simulink model "ac3_example_MMCT"  (R2023a)
settings: Solver=FixedStepDiscrete  StartTime=0.0  StopTime=3  FixedStep=Ts  RelTol=1e-3  EnableMultiTasking=on
PreLoadFcn:
  | Ts = 2e-6;
undefined symbols (not defined in the file): DiscIntNeverNeededParam
libraries: simulink_extras x7, spsCurrentMeasurementLib x3, spsVoltageMeasurementLib x3, spsDrivesPrivateModels x2, spsStairGeneratorLib x2, spsThreePhaseSourceLib x1, spsDrivesDcBusModel x1, spsSpaceVectorModulatorLib x1, eeAdaptiveController x1, slctrlblks x1, simulink x1, slpidlib x1
(part 3 of 3)

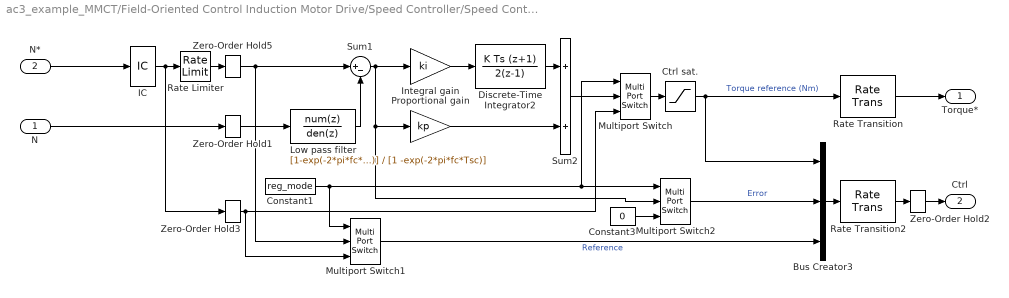
== system ac3_example_MMCT/Field-Oriented Control Induction Motor Drive/Speed Controller/Speed Controller (AC)/AC678/AC678 ==
  N : Inport
  N* : Inport  Port=2
  Bus Creator3 : BusCreator  Inputs=3
  Constant1 : Constant  Value=reg_mode
  Constant3 : Constant  Value=0
  Ctrl sat. : Saturate  UpperLimit=ctrl_sat(2)  LowerLimit=ctrl_sat(1)
  Discrete-Time Integrator2 : DiscreteIntegrator  IntegratorMethod=Integration: Trapezoidal  SampleTime=Tsc  LimitOutput=on  UpperSaturationLimit=ctrl_sat(2)  LowerSaturationLimit=ctrl_sat(1)  ICPrevOutput=DiscIntNeverNeededParam  ICPrevScaledInput=DiscIntNeverNeededParam
  IC : InitialCondition  Value=0
  Integral gain : Gain  Gain=ki  SaturateOnIntegerOverflow=on  OutDataTypeStr=Inherit: Same as input  ParamDataTypeStr=Inherit: Same as input
  Low pass filter : DiscreteTransferFcn  Numerator=[1-exp(-2*pi*fc*Tsc)]  Denominator=[1 -exp(-2*pi*fc*Tsc)]  SampleTime=Tsc
  Multiport Switch : MultiPortSwitch  Inputs=2  InputSameDT=off
  Multiport Switch1 : MultiPortSwitch  Inputs=2  InputSameDT=off
  Multiport Switch2 : MultiPortSwitch  Inputs=2  InputSameDT=off
  Proportional gain : Gain  Gain=kp  SaturateOnIntegerOverflow=on  OutDataTypeStr=Inherit: Same as input  ParamDataTypeStr=Inherit: Same as input
  Rate Limiter : RateLimiter  RisingSlewLimit=ramp(2)  FallingSlewLimit=ramp(1)  SampleTimeMode=inherited  LinearizeAsGain=off
  Rate Transition : RateTransition
  Rate Transition2 : RateTransition
  Sum1 : Sum  Inputs=|+-  InputSameDT=on  SaturateOnIntegerOverflow=on  OutDataTypeStr=Inherit: Same as first input
  Sum2 : Sum  InputSameDT=on  SaturateOnIntegerOverflow=on  OutDataTypeStr=Inherit: Same as first input
  Zero-Order Hold1 : ZeroOrderHold  SampleTime=Tsc
  Zero-Order Hold2 : ZeroOrderHold  SampleTime=Ts
  Zero-Order Hold3 : ZeroOrderHold  SampleTime=Tsc
  Zero-Order Hold5 : ZeroOrderHold  SampleTime=Tsc
  Torque* : Outport  VectorParamsAs1DForOutWhenUnconnected=off
  Ctrl : Outport  Port=2  VectorParamsAs1DForOutWhenUnconnected=off
  wires:
  N/1 -> Zero-Order Hold1/1
  N*/1 -> IC/1
  Ctrl sat./1 -> Rate Transition/1, Bus Creator3/1  "Torque reference (Nm)"
  Integral gain/1 -> Discrete-Time Integrator2/1
  Sum1/1 -> Integral gain/1, Proportional gain/1, Multiport Switch2/2
  Discrete-Time Integrator2/1 -> Sum2/1
  Proportional gain/1 -> Sum2/2
  Rate Transition/1 -> Torque*/1
  IC/1 -> Rate Limiter/1, Zero-Order Hold3/1
  Zero-Order Hold1/1 -> Low pass filter/1
  Rate Transition2/1 -> Zero-Order Hold2/1
  Bus Creator3/1 -> Rate Transition2/1
  Zero-Order Hold2/1 -> Ctrl/1
  Low pass filter/1 -> Sum1/2
  Rate Limiter/1 -> Zero-Order Hold5/1
  Zero-Order Hold5/1 -> Sum1/1, Multiport Switch1/2
  Multiport Switch/1 -> Ctrl sat./1
  Constant1/1 -> Multiport Switch2/1, Multiport Switch/1, Multiport Switch1/1
  Sum2/1 -> Multiport Switch/2
  Zero-Order Hold3/1 -> Multiport Switch/3, Multiport Switch1/3
  Multiport Switch1/1 -> Bus Creator3/3  "Reference"
  Multiport Switch2/1 -> Bus Creator3/2  "Error"
  Constant3/1 -> Multiport Switch2/3

== system ac3_example_MMCT/Field-Oriented Control Induction Motor Drive/F.O.C./Detailed/Switching control/Control 1-2/Subsystem1 ==
  Sig : Inport
  Constant : Constant
  Constant1 : Constant  Value=freq_max
  Discrete-Time Integrator : DiscreteIntegrator  IntegratorMethod=Integration: Trapezoidal  ExternalReset=rising  SampleTime=Tvect  ICPrevOutput=DiscIntNeverNeededParam  ICPrevScaledInput=DiscIntNeverNeededParam
  Relational Operator : RelationalOperator  ZeroCross=off  InputSameDT=off
  Unit Delay : UnitDelay  SampleTime=Tvect  HasFrameUpgradeWarning=on
  Trig : Outport  VectorParamsAs1DForOutWhenUnconnected=off
  wires:
  Constant1/1 -> Discrete-Time Integrator/1
  Constant/1 -> Relational Operator/2
  Discrete-Time Integrator/1 -> Relational Operator/1
  Relational Operator/1 -> Unit Delay/1
  Sig/1 -> Discrete-Time Integrator/2
  Unit Delay/1 -> Trig/1

== system ac3_example_MMCT/Field-Oriented Control Induction Motor Drive/F.O.C./Detailed/Switching control/Control 1-2/Subsystem3 ==
  Sig : Inport
  Constant : Constant
  Constant1 : Constant  Value=freq_max
  Discrete-Time Integrator : DiscreteIntegrator  IntegratorMethod=Integration: Trapezoidal  ExternalReset=rising  SampleTime=Tvect  ICPrevOutput=DiscIntNeverNeededParam  ICPrevScaledInput=DiscIntNeverNeededParam
  Relational Operator : RelationalOperator  ZeroCross=off  InputSameDT=off
  Unit Delay : UnitDelay  SampleTime=Tvect  HasFrameUpgradeWarning=on
  Trig : Outport  VectorParamsAs1DForOutWhenUnconnected=off
  wires:
  Unit Delay/1 -> Trig/1
  Sig/1 -> Discrete-Time Integrator/2
  Relational Operator/1 -> Unit Delay/1
  Discrete-Time Integrator/1 -> Relational Operator/1
  Constant/1 -> Relational Operator/2
  Constant1/1 -> Discrete-Time Integrator/1

== system ac3_example_MMCT/Field-Oriented Control Induction Motor Drive/F.O.C./Detailed/Switching control/Control 3-4/Subsystem1 ==
  Sig : Inport
  Constant : Constant
  Constant1 : Constant  Value=freq_max
  Discrete-Time Integrator : DiscreteIntegrator  IntegratorMethod=Integration: Trapezoidal  ExternalReset=rising  SampleTime=Tvect  ICPrevOutput=DiscIntNeverNeededParam  ICPrevScaledInput=DiscIntNeverNeededParam
  Relational Operator : RelationalOperator  ZeroCross=off  InputSameDT=off
  Unit Delay : UnitDelay  SampleTime=Tvect  HasFrameUpgradeWarning=on
  Trig : Outport  VectorParamsAs1DForOutWhenUnconnected=off
  wires:
  Unit Delay/1 -> Trig/1
  Sig/1 -> Discrete-Time Integrator/2
  Relational Operator/1 -> Unit Delay/1
  Discrete-Time Integrator/1 -> Relational Operator/1
  Constant/1 -> Relational Operator/2
  Constant1/1 -> Discrete-Time Integrator/1

== system ac3_example_MMCT/Field-Oriented Control Induction Motor Drive/F.O.C./Detailed/Switching control/Control 3-4/Subsystem3 ==
  Sig : Inport
  Constant : Constant
  Constant1 : Constant  Value=freq_max
  Discrete-Time Integrator : DiscreteIntegrator  IntegratorMethod=Integration: Trapezoidal  ExternalReset=rising  SampleTime=Tvect  ICPrevOutput=DiscIntNeverNeededParam  ICPrevScaledInput=DiscIntNeverNeededParam
  Relational Operator : RelationalOperator  ZeroCross=off  InputSameDT=off
  Unit Delay : UnitDelay  SampleTime=Tvect  HasFrameUpgradeWarning=on
  Trig : Outport  VectorParamsAs1DForOutWhenUnconnected=off
  wires:
  Constant1/1 -> Discrete-Time Integrator/1
  Constant/1 -> Relational Operator/2
  Discrete-Time Integrator/1 -> Relational Operator/1
  Relational Operator/1 -> Unit Delay/1
  Sig/1 -> Discrete-Time Integrator/2
  Unit Delay/1 -> Trig/1

== system ac3_example_MMCT/Field-Oriented Control Induction Motor Drive/F.O.C./Detailed/Switching control/Control 5-6/Subsystem1 ==
  Sig : Inport
  Constant : Constant
  Constant1 : Constant  Value=freq_max
  Discrete-Time Integrator : DiscreteIntegrator  IntegratorMethod=Integration: Trapezoidal  ExternalReset=rising  SampleTime=Tvect  ICPrevOutput=DiscIntNeverNeededParam  ICPrevScaledInput=DiscIntNeverNeededParam
  Relational Operator : RelationalOperator  ZeroCross=off  InputSameDT=off
  Unit Delay : UnitDelay  SampleTime=Tvect  HasFrameUpgradeWarning=on
  Trig : Outport  VectorParamsAs1DForOutWhenUnconnected=off
  wires:
  Constant1/1 -> Discrete-Time Integrator/1
  Constant/1 -> Relational Operator/2
  Discrete-Time Integrator/1 -> Relational Operator/1
  Relational Operator/1 -> Unit Delay/1
  Sig/1 -> Discrete-Time Integrator/2
  Unit Delay/1 -> Trig/1

== system ac3_example_MMCT/Field-Oriented Control Induction Motor Drive/F.O.C./Detailed/Switching control/Control 5-6/Subsystem3 ==
  Sig : Inport
  Constant : Constant
  Constant1 : Constant  Value=freq_max
  Discrete-Time Integrator : DiscreteIntegrator  IntegratorMethod=Integration: Trapezoidal  ExternalReset=rising  SampleTime=Tvect  ICPrevOutput=DiscIntNeverNeededParam  ICPrevScaledInput=DiscIntNeverNeededParam
  Relational Operator : RelationalOperator  ZeroCross=off  InputSameDT=off
  Unit Delay : UnitDelay  SampleTime=Tvect  HasFrameUpgradeWarning=on
  Trig : Outport  VectorParamsAs1DForOutWhenUnconnected=off
  wires:
  Unit Delay/1 -> Trig/1
  Sig/1 -> Discrete-Time Integrator/2
  Relational Operator/1 -> Unit Delay/1
  Discrete-Time Integrator/1 -> Relational Operator/1
  Constant/1 -> Relational Operator/2
  Constant1/1 -> Discrete-Time Integrator/1

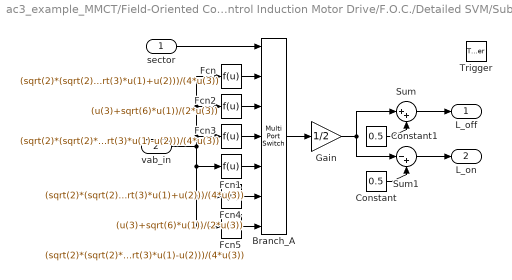
== system ac3_example_MMCT/Field-Oriented Control Induction Motor Drive/F.O.C./Detailed SVM/Subsystem1/switching time calculator/switching_timing BrA ==
  sector : Inport
  vab_in : Inport  Port=2
  Trigger : TriggerPort  VariantControl=Variant
  Branch_A : MultiPortSwitch  Inputs=6
  Constant : Constant  Value=0.5
  Constant1 : Constant  Value=0.5
  Fcn : Fcn  Expr=(sqrt(2)*(sqrt(2)*u(3)+sqrt(3)*u(1)+u(2)))/(4*u(3))
  Fcn1 : Fcn  Expr=(sqrt(2)*(sqrt(2)*u(3)+sqrt(3)*u(1)+u(2)))/(4*u(3))
  Fcn2 : Fcn  Expr=(u(3)+sqrt(6)*u(1))/(2*u(3))
  Fcn3 : Fcn  Expr=(sqrt(2)*(sqrt(2)*u(3)+sqrt(3)*u(1)-u(2)))/(4*u(3))
  Fcn4 : Fcn  Expr=(u(3)+sqrt(6)*u(1))/(2*u(3))
  Fcn5 : Fcn  Expr=(sqrt(2)*(sqrt(2)*u(3)+sqrt(3)*u(1)-u(2)))/(4*u(3))
  Gain : Gain  Gain=1/2  SaturateOnIntegerOverflow=on  OutDataTypeStr=Inherit: Same as input  ParamDataTypeStr=Inherit: Same as input
  Sum : Sum  Inputs=|++  InputSameDT=on  SaturateOnIntegerOverflow=on  OutDataTypeStr=Inherit: Same as first input
  Sum1 : Sum  Inputs=|-+  InputSameDT=on  SaturateOnIntegerOverflow=on  OutDataTypeStr=Inherit: Same as first input
  L_off : Outport  VectorParamsAs1DForOutWhenUnconnected=off
  L_on : Outport  Port=2  VectorParamsAs1DForOutWhenUnconnected=off
  wires:
  Fcn/1 -> Branch_A/2
  Fcn2/1 -> Branch_A/3
  Fcn3/1 -> Branch_A/4
  Fcn1/1 -> Branch_A/5
  Fcn4/1 -> Branch_A/6
  Fcn5/1 -> Branch_A/7
  Branch_A/1 -> Gain/1
  Gain/1 -> Sum/1, Sum1/1
  Constant/1 -> Sum1/2
  Constant1/1 -> Sum/2
  Sum/1 -> L_off/1
  Sum1/1 -> L_on/1
  sector/1 -> Branch_A/1
  vab_in/1 -> Fcn3/1, Fcn2/1, Fcn/1, Fcn1/1, Fcn4/1, Fcn5/1

== system ac3_example_MMCT/Field-Oriented Control Induction Motor Drive/F.O.C./Detailed SVM/Subsystem1/switching time calculator/switching_timing BrB ==
  sector : Inport
  Vab_inp : Inport  Port=2
  Trigger : TriggerPort  VariantControl=Variant
  Branch_B : MultiPortSwitch  Inputs=6
  Constant : Constant  Value=0.5
  Constant1 : Constant  Value=0.5
  Fcn10 : Fcn  Expr=(u(3)+sqrt(2)*u(2))/(2*u(3))
  Fcn11 : Fcn  Expr=(sqrt(2)*(sqrt(2)*u(3)-sqrt(3)*u(1)+u(2)))/(4*u(3))
  Fcn6 : Fcn  Expr=(sqrt(2)*(sqrt(2)*u(3)-sqrt(3)*u(1)+3*u(2)))/(4*u(3))
  Fcn7 : Fcn  Expr=(sqrt(2)*(sqrt(2)*u(3)-sqrt(3)*u(1)+3*u(2)))/(4*u(3))
  Fcn8 : Fcn  Expr=(u(3)+sqrt(2)*u(2))/(2*u(3))
  Fcn9 : Fcn  Expr=(sqrt(2)*(sqrt(2)*u(3)-sqrt(3)*u(1)+u(2)))/(4*u(3))
  Gain : Gain  Gain=1/2  SaturateOnIntegerOverflow=on  OutDataTypeStr=Inherit: Same as input  ParamDataTypeStr=Inherit: Same as input
  Sum : Sum  Inputs=|++  InputSameDT=on  SaturateOnIntegerOverflow=on  OutDataTypeStr=Inherit: Same as first input
  Sum1 : Sum  Inputs=|-+  InputSameDT=on  SaturateOnIntegerOverflow=on  OutDataTypeStr=Inherit: Same as first input
  L_off : Outport  VectorParamsAs1DForOutWhenUnconnected=off
  L_on : Outport  Port=2  VectorParamsAs1DForOutWhenUnconnected=off
  wires:
  sector/1 -> Branch_B/1
  Sum1/1 -> L_on/1
  Sum/1 -> L_off/1
  Constant1/1 -> Sum/2
  Constant/1 -> Sum1/2
  Gain/1 -> Sum1/1, Sum/1
  Branch_B/1 -> Gain/1
  Vab_inp/1 -> Fcn10/1, Fcn11/1, Fcn7/1, Fcn8/1, Fcn6/1, Fcn9/1
  Fcn7/1 -> Branch_B/5
  Fcn8/1 -> Branch_B/3
  Fcn6/1 -> Branch_B/2
  Fcn9/1 -> Branch_B/4
  Fcn10/1 -> Branch_B/6
  Fcn11/1 -> Branch_B/7

== system ac3_example_MMCT/Field-Oriented Control Induction Motor Drive/F.O.C./Detailed SVM/Subsystem1/switching time calculator/switching_timing BrC ==
  sector : Inport
  Vab_inp : Inport  Port=2
  Trigger : TriggerPort  VariantControl=Variant
  Branch_C : MultiPortSwitch  Inputs=6
  Constant : Constant  Value=0.5
  Constant1 : Constant  Value=0.5
  Fcn12 : Fcn  Expr=(u(3)-sqrt(2)*u(2))/(2*u(3))
  Fcn13 : Fcn  Expr=(sqrt(2)*(sqrt(2)*u(3)-sqrt(3)*u(1)-3*u(2)))/(4*u(3))
  Fcn14 : Fcn  Expr=(sqrt(2)*(sqrt(2)*u(3)-sqrt(3)*u(1)-u(2)))/(4*u(3))
  Fcn15 : Fcn  Expr=(sqrt(2)*(sqrt(2)*u(3)-sqrt(3)*u(1)-u(2)))/(4*u(3))
  Fcn16 : Fcn  Expr=(u(3)-sqrt(2)*u(2))/(2*u(3))
  Fcn17 : Fcn  Expr=(sqrt(2)*(sqrt(2)*u(3)-sqrt(3)*u(1)-3*u(2)))/(4*u(3))
  Gain : Gain  Gain=1/2  SaturateOnIntegerOverflow=on  OutDataTypeStr=Inherit: Same as input  ParamDataTypeStr=Inherit: Same as input
  Sum : Sum  Inputs=|++  InputSameDT=on  SaturateOnIntegerOverflow=on  OutDataTypeStr=Inherit: Same as first input
  Sum1 : Sum  Inputs=|-+  InputSameDT=on  SaturateOnIntegerOverflow=on  OutDataTypeStr=Inherit: Same as first input
  L_off : Outport  VectorParamsAs1DForOutWhenUnconnected=off
  L_on : Outport  Port=2  VectorParamsAs1DForOutWhenUnconnected=off
  wires:
  Vab_inp/1 -> Fcn16/1, Fcn14/1, Fcn12/1, Fcn13/1, Fcn15/1, Fcn17/1
  Branch_C/1 -> Gain/1
  Gain/1 -> Sum/1, Sum1/1
  Constant/1 -> Sum1/2
  Constant1/1 -> Sum/2
  Sum/1 -> L_off/1
  Sum1/1 -> L_on/1
  Fcn15/1 -> Branch_C/5
  Fcn16/1 -> Branch_C/3
  Fcn14/1 -> Branch_C/2
  Fcn17/1 -> Branch_C/4
  Fcn12/1 -> Branch_C/6
  Fcn13/1 -> Branch_C/7
  sector/1 -> Branch_C/1

== matlab function ac3_example_MMCT/Field-Oriented Control Induction Motor Drive/MATLAB Function ==
  data: u input; y output
function y = fcn(u)
y=u;
coder.extrinsic("set_param");
if (0.55<u)&&(u<3)
    if u<0.65
    set_param('ac3_example_MMCT/Sine_Wave','Amplitude','4')
    set_param('ac3_example_MMCT/Sine_Wave','Frequency','10')
    elseif (0.65<u)&&(u<1.25)
            set_param('ac3_example_MMCT/Sine_Wave','Amplitude','5')
            set_param('ac3_example_MMCT/Sine_Wave','Frequency','1')
    elseif (1.25<u)&&(u<2.25)
                   set_param('ac3_example_MMCT/Sine_Wave','Amplitude','3')
                   set_param('ac3_example_MMCT/Sine_Wave','Frequency','5')
    
else
  set_param('ac3_example_MMCT/Sine_Wave','Amplitude','2')    
  set_param('ac3_example_MMCT/Sine_Wave','Frequency','20')
    end
end

== matlab function ac3_example_MMCT/Field-Oriented Control Induction Motor Drive/MATLAB Function1 ==
  data: u input; y output
function y = fcn(u)
y=u;
coder.extrinsic("set_param");
% Llr=0.0003027;
x=u+9.295e-3;
 set_param('ac3_example_MMCT/Field-Oriented Control Induction Motor Drive','Rr','1');
